simulink model "TF_1"  (R2015a)
settings: Solver=ode45  StartTime=0.0  StopTime=60  RelTol=1e-3
values from neighbouring files (symbols this model uses):
  b = 200    [matlabparachot.mat]    (also in with_TF_1.m = 0.1)
  k = 0.1    [with_TF_1.m]
  m = 1    [with_TF_1.m]
settings Model: Creator=ahmed alaa  LastModifiedBy=ahmed alaa

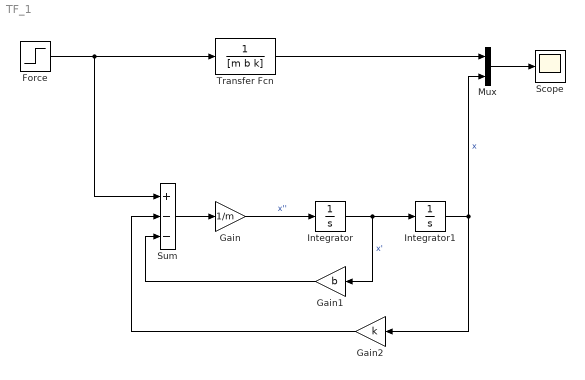
== system TF_1 ==
  Force : Step  After=9.8*m  SampleTime=0
  Gain : Gain  Gain=1/m
  Gain1 : Gain  Gain=b
  Gain2 : Gain  Gain=k
  Integrator : Integrator
  Integrator1 : Integrator
  Mux : Mux  Inputs=2
  Scope : Scope
  Sum : Sum  Inputs=+--
  Transfer Fcn : TransferFcn  Denominator=[m b k]
  wires:
  Force/1 -> Sum/1, Transfer Fcn/1
  Mux/1 -> Scope/1
  Sum/1 -> Gain/1
  Gain/1 -> Integrator/1  "x''"
  Integrator/1 -> Integrator1/1, Gain1/1  "x'"
  Integrator1/1 -> Mux/2, Gain2/1  "x"
  Gain1/1 -> Sum/3
  Gain2/1 -> Sum/2
  Transfer Fcn/1 -> Mux/1
